simulink model "trainn_traction_system_4motors_CRH3_ver1"  (R2020b)
settings: Solver=VariableStepAuto  StartTime=0.0  StopTime=3  RelTol=1e-3
model workspace (MAT data in the model file):
  C = 0.016
  J = 5
  L = 0.005
  Llr = 0.006
  Lls = 0.001416
  Lm = 0.0254
  R = 0.2
  Rr = 0.16
  Rs = 0.15
  T = 1e-06
  Tloadmax = 100
  Tloadstart = 2
  Tpwm = 0.0001
  Ts = 0.0008
  Vdc_ref = 2700
  Vpeak = 1550
  f = 50
  noiseDense = 0.01
  np = 2
  sample_time = 2e-05
  tE1 = 3.25
  tE1w = 10
  tE2 = 10
  tE2w = 10
  tE3 = 10
  tE3w = 10
  tE4 = 10
  tE4w = 10
  t_precharge = 0.15
  w = 314.159265359
libraries: powerlib x19, simulink x19, pid_lib x1, eeSinusoidalMeasurementV2 x1
(part 2 of 3)

== system trainn_traction_system_4motors_CRH3_ver1/motor module2/Subsystem2/转矩调节器ATR ==
  " " : Inport
  Integrator : Integrator
  I积分放大倍数 : Gain  Gain=1.1
  PI输出限幅1 : Saturate  UpperLimit=600  LowerLimit=-600
  P比例放大倍数 : Gain  Gain=1.6
  Scope : Scope  NumInputPorts=2
  Sum3 : Sum  Inputs=|++
  带限幅的连续积分1 : Integrator  LimitOutput=on  UpperSaturationLimit=65  LowerSaturationLimit=-65
  ist* : Outport  VectorParamsAs1DForOutWhenUnconnected=off
  wires:
  " "/1 -> I积分放大倍数/1, P比例放大倍数/1
  I积分放大倍数/1 -> Integrator/1
  Sum3/1 -> PI输出限幅1/1
  P比例放大倍数/1 -> Sum3/1
  Integrator/1 -> Scope/2, Sum3/2
  PI输出限幅1/1 -> Scope/1, ist*/1

== system trainn_traction_system_4motors_CRH3_ver1/motor module2/Subsystem2/转速调节器ASR ==
  "  " : Inport
  Integrator : Integrator
  I积分放大倍数 : Gain  Gain=0.08
  PI输出限幅2 : Saturate  UpperLimit=400  LowerLimit=-400
  P比例放大倍数 : Gain  Gain=12
  Scope : Scope  NumInputPorts=2
  Sum1 : Sum  Inputs=|++
  带限幅的连续积分1 : Integrator  LimitOutput=on  UpperSaturationLimit=80  LowerSaturationLimit=-80
  Te* : Outport  VectorParamsAs1DForOutWhenUnconnected=off
  wires:
  I积分放大倍数/1 -> Integrator/1
  "  "/1 -> I积分放大倍数/1, P比例放大倍数/1
  P比例放大倍数/1 -> Sum1/1
  Integrator/1 -> Scope/2, Sum1/2
  Sum1/1 -> PI输出限幅2/1
  PI输出限幅2/1 -> Scope/1, Te*/1

== system trainn_traction_system_4motors_CRH3_ver1/motor module3/Subsystem3/ACMR ==
  "  " : Inport
  Integrator : Integrator
  I积分放大倍数 : Gain  Gain=50
  PI输出限幅 : Saturate  UpperLimit=Vdc_ref/sqrt(6)  LowerLimit=-Vdc_ref/sqrt(6)
  P比例放大倍数 : Gain
  Scope : Scope  NumInputPorts=2
  Sum1 : Sum  Inputs=|++
  带限幅的连续积分1 : Integrator  LimitOutput=on  UpperSaturationLimit=390  LowerSaturationLimit=-390
  " " : Outport  VectorParamsAs1DForOutWhenUnconnected=off
  wires:
  Sum1/1 -> PI输出限幅/1
  PI输出限幅/1 -> " "/1, Scope/1
  P比例放大倍数/1 -> Sum1/1
  I积分放大倍数/1 -> Integrator/1
  "  "/1 -> I积分放大倍数/1, P比例放大倍数/1
  Integrator/1 -> Scope/2, Sum1/2

== system trainn_traction_system_4motors_CRH3_ver1/motor module3/Subsystem3/ACTR ==
  "  " : Inport
  Integrator : Integrator
  I积分放大倍数 : Gain  Gain=3.5
  PI输出限幅 : Saturate  UpperLimit=Vdc_ref/sqrt(6)  LowerLimit=-1*Vdc_ref/sqrt(6)
  PI输出限幅1 : Saturate  UpperLimit=Vdc_ref  LowerLimit=-1*Vdc_ref
  P比例放大倍数 : Gain  Gain=1.5
  Scope : Scope  NumInputPorts=2
  Sum1 : Sum  Inputs=|++
  带限幅的连续积分1 : Integrator  LimitOutput=on  UpperSaturationLimit=400  LowerSaturationLimit=-400
  " " : Outport  VectorParamsAs1DForOutWhenUnconnected=off
  wires:
  Sum1/1 -> PI输出限幅/1
  PI输出限幅/1 -> " "/1, Scope/1
  P比例放大倍数/1 -> Sum1/1
  I积分放大倍数/1 -> Integrator/1
  "  "/1 -> I积分放大倍数/1, P比例放大倍数/1
  Integrator/1 -> Scope/2, Sum1/2

== system trainn_traction_system_4motors_CRH3_ver1/motor module3/Subsystem3/SVPWM ==
  Udc : Inport
  Ualpha : Inport  Port=2
  Ubeta : Inport  Port=3
  " Gen Gate" : MATLAB Function  TreatAsAtomicUnit=on
  Clock : Clock
  Constant2 : Constant  Value=Ts
  Constant3 : Constant  Value=Ts
  Data Type Conversion : DataTypeConversion  OutDataTypeStr=boolean
  Delay{,1..4} (5 alike) : Delay  DelayLength=1  InitialCondition=0
  MATLAB Function1 : MATLAB Function  TreatAsAtomicUnit=on
  MATLAB Function3 : MATLAB Function  TreatAsAtomicUnit=on
  Pulse Generator : DiscretePulseGenerator  PulseType=Time based  Period=Ts
  Scope1 : Scope  NumInputPorts=3
  Scope3 : Scope
  find section1 : Subsystem
  g : Outport
  wires:
  Ualpha/1 -> find section1/1(Ualpha), MATLAB Function3/2(Ualpha)
  Pulse Generator/1 -> Data Type Conversion/1
  MATLAB Function1/2(newT0) -> " Gen Gate"/4(T0), Delay/1
  Delay1/1 -> MATLAB Function1/1(old_t0)
  MATLAB Function3/3(T2) -> Scope1/3, MATLAB Function1/6(T2)
  Ubeta/1 -> find section1/2(Ubeta), MATLAB Function3/3(Ubeta)
  find section1/1(section) -> MATLAB Function1/7(sec), MATLAB Function3/5(sec)
  Constant2/1 -> MATLAB Function3/4(Ts)
  MATLAB Function3/2(T1) -> Scope1/2, MATLAB Function1/5(T1)
  MATLAB Function1/1(new_t0) -> Scope3/1, Delay1/1, " Gen Gate"/2(t0)
  Clock/1 -> " Gen Gate"/1(t), MATLAB Function1/2(t)
  MATLAB Function3/1(T0) -> MATLAB Function1/4(T0), Scope1/1
  Constant3/1 -> " Gen Gate"/3(Ts)
  Udc/1 -> MATLAB Function3/1(Udc)
  " Gen Gate"/1(g) -> g/1
  Data Type Conversion/1 -> MATLAB Function1/3(trigger)
  MATLAB Function1/5(newSec) -> Delay2/1, " Gen Gate"/7(sec)
  Delay2/1 -> MATLAB Function1/11(oldSec)
  MATLAB Function1/4(newT2) -> Delay3/1, " Gen Gate"/6(T2)
  Delay3/1 -> MATLAB Function1/10(oldT2)
  MATLAB Function1/3(newT1) -> Delay4/1, " Gen Gate"/5(T1)
  Delay4/1 -> MATLAB Function1/9(oldT1)
  Delay/1 -> MATLAB Function1/8(oldT0)

== system trainn_traction_system_4motors_CRH3_ver1/motor module3/Subsystem3/SVPWM1 ==
  Udc : Inport
  Ualpha : Inport  Port=2
  Ubeta : Inport  Port=3
  Constant2 : Constant  Value=Tpwm
  Constant4 : Constant  Value=Tpwm
  MATLAB Function10 : MATLAB Function  TreatAsAtomicUnit=on
  MATLAB Function3 : MATLAB Function  TreatAsAtomicUnit=on
  Mux : Mux  Inputs=6
  Repeating Sequence1 : simulink/Sources/Repeating Sequence  rep_seq_t=[0 Tpwm]  rep_seq_y=[0 Tpwm]
  Scope1 : Scope  NumInputPorts=3
  find section1 : Subsystem
  g : Outport
  wires:
  Ualpha/1 -> find section1/1(Ualpha), MATLAB Function3/2(Ualpha)
  Ubeta/1 -> find section1/2(Ubeta), MATLAB Function3/3(Ubeta)
  Constant2/1 -> MATLAB Function3/4(Ts)
  MATLAB Function3/1(T0) -> Scope1/1
  Udc/1 -> MATLAB Function3/1(Udc)
  MATLAB Function3/2(T1) -> Scope1/2, MATLAB Function10/1(Ta)
  find section1/1(section) -> MATLAB Function10/4(section), MATLAB Function3/5(sec)
  Constant4/1 -> MATLAB Function10/3(Tpwm)
  Repeating Sequence1/1 -> MATLAB Function10/5(t)
  MATLAB Function3/3(T2) -> Scope1/3, MATLAB Function10/2(Tb)
  MATLAB Function10/6(gCN) -> Mux/6
  MATLAB Function10/5(gC) -> Mux/5
  MATLAB Function10/4(gBN) -> Mux/4
  MATLAB Function10/3(gB) -> Mux/3
  MATLAB Function10/2(gAN) -> Mux/2
  MATLAB Function10/1(gA) -> Mux/1
  Mux/1 -> g/1

== system trainn_traction_system_4motors_CRH3_ver1/motor module3/Subsystem3/Subsystem ==
  note: Tr = Lr / Rr
  note: phy_r
  note: ws
  note: w1
  id(im) : Inport
  iq(it) : Inport  Port=2
  w : Inport  Port=3
  Divide{,2..4} (4 alike) : Product  Inputs=/*
  Divide1 : Product  Inputs=*/
  Gain1 : Gain  Gain=Lm
  Gain2 : Gain  Gain=Lm
  Integrator1 : Integrator  InitialCondition=1e-5
  Integrator2 : Integrator
  Lr : Constant  Value=Llr + 1.5*Lm
  Rr : Constant  Value=Rr
  Scope3 : Scope  NumInputPorts=2
  Sum : Sum  Inputs=-+|
  Sum1 : Sum  Inputs=|++
  phi : Outport
  theta : Outport  Port=2
  wires:
  Divide/1 -> Sum1/1
  Divide3/1 -> Divide/2
  Sum/1 -> Integrator1/1
  iq(it)/1 -> Gain2/1, Scope3/2
  Sum1/1 -> Integrator2/1
  id(im)/1 -> Gain1/1, Scope3/1
  w/1 -> Sum1/2
  Integrator2/1 -> theta/1
  Lr/1 -> Divide1/1
  Rr/1 -> Divide1/2
  Divide2/1 -> Sum/2
  Gain1/1 -> Divide2/2
  Integrator1/1 -> Divide4/2, Divide/1, phi/1
  Divide4/1 -> Sum/1
  Divide1/1 -> Divide3/1, Divide2/1, Divide4/1
  Gain2/1 -> Divide3/2

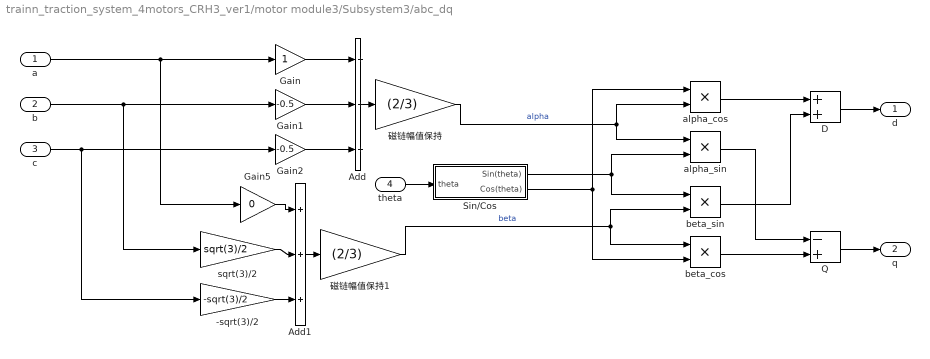
== system trainn_traction_system_4motors_CRH3_ver1/motor module3/Subsystem3/abc_dq ==
  a : Inport
  b : Inport  Port=2
  c : Inport  Port=3
  theta : Inport  Port=4
  -sqrt(3)/2 : Gain  Gain=-sqrt(3)/2
  Add : Sum  Inputs=3
  Add1 : Sum  Inputs=3
  D : Sum
  Gain : Gain
  Gain1 : Gain  Gain=-0.5
  Gain2 : Gain  Gain=-0.5
  Gain5 : Gain  Gain=0
  Q : Sum  Inputs=-+
  Sin/Cos : Subsystem
  alpha_cos : Product
  alpha_sin : Product
  beta_cos : Product
  beta_sin : Product
  sqrt(3)/2 : Gain  Gain=sqrt(3)/2
  磁链幅值保持 : Gain  Gain=(2/3)
  磁链幅值保持1 : Gain  Gain=(2/3)
  d : Outport  VectorParamsAs1DForOutWhenUnconnected=off
  q : Outport  Port=2  VectorParamsAs1DForOutWhenUnconnected=off
  wires:
  磁链幅值保持1/1 -> beta_cos/1, beta_sin/2  "beta"
  D/1 -> d/1
  Sin/Cos/2(Cos(theta)) -> beta_cos/2, alpha_cos/1
  alpha_sin/1 -> Q/1
  Q/1 -> q/1
  beta_sin/1 -> D/2
  beta_cos/1 -> Q/2
  Sin/Cos/1(Sin(theta)) -> beta_sin/1, alpha_sin/2
  磁链幅值保持/1 -> alpha_cos/2, alpha_sin/1  "alpha"
  Add1/1 -> 磁链幅值保持1/1
  c/1 -> Gain2/1, -sqrt(3)/2/1
  a/1 -> Gain5/1, Gain/1
  Gain2/1 -> Add/3
  sqrt(3)/2/1 -> Add1/2
  theta/1 -> Sin/Cos/1(theta)
  b/1 -> sqrt(3)/2/1, Gain1/1
  -sqrt(3)/2/1 -> Add1/3
  Gain1/1 -> Add/2
  Gain5/1 -> Add1/1
  alpha_cos/1 -> D/1
  Add/1 -> 磁链幅值保持/1
  Gain/1 -> Add/1

== system trainn_traction_system_4motors_CRH3_ver1/motor module3/Subsystem3/dq-alpha\beta1 ==
  Q : Inport
  D : Inport  Port=2
  theta : Inport  Port=3
  Product{,1..3} (4 alike) : Product
  Sum1 : Sum  Inputs=++|
  Sum3 : Sum  Inputs=|+-
  Trigonometric Function : Trigonometry
  Trigonometric Function1 : Trigonometry  Operator=cos
  alpha : Outport
  beta : Outport  Port=2
  wires:
  Sum1/1 -> beta/1
  Product3/1 -> Sum1/2
  Product2/1 -> Sum1/1
  Sum3/1 -> alpha/1
  Product1/1 -> Sum3/2
  Product/1 -> Sum3/1
  Trigonometric Function/1 -> Product1/1, Product2/1
  Trigonometric Function1/1 -> Product/2, Product3/1
  Q/1 -> Product1/2, Product3/2
  theta/1 -> Trigonometric Function/1, Trigonometric Function1/1
  D/1 -> Product2/2, Product/1

== system trainn_traction_system_4motors_CRH3_ver1/motor module3/Subsystem3/磁链调节器APhirR ==
  " " : Inport
  Integrator : Integrator
  I积分放大倍数 : Gain  Gain=3.6
  PI输出限幅1 : Saturate  UpperLimit=13  LowerLimit=-13
  P比例放大倍数 : Gain  Gain=1.8
  Scope : Scope  NumInputPorts=2
  Sum1 : Sum  Inputs=|++
  带限幅的连续积分1 : Integrator  LimitOutput=on  UpperSaturationLimit=15  LowerSaturationLimit=-15
  ism* : Outport  VectorParamsAs1DForOutWhenUnconnected=off
  wires:
  P比例放大倍数/1 -> Sum1/1
  " "/1 -> I积分放大倍数/1, P比例放大倍数/1
  Sum1/1 -> ism*/1, Scope/1
  I积分放大倍数/1 -> Integrator/1
  Integrator/1 -> Scope/2, Sum1/2

== system trainn_traction_system_4motors_CRH3_ver1/motor module3/Subsystem3/转矩调节器ATR ==
  " " : Inport
  Integrator : Integrator
  I积分放大倍数 : Gain  Gain=1.1
  PI输出限幅1 : Saturate  UpperLimit=600  LowerLimit=-600
  P比例放大倍数 : Gain  Gain=1.6
  Scope : Scope  NumInputPorts=2
  Sum3 : Sum  Inputs=|++
  带限幅的连续积分1 : Integrator  LimitOutput=on  UpperSaturationLimit=65  LowerSaturationLimit=-65
  ist* : Outport  VectorParamsAs1DForOutWhenUnconnected=off
  wires:
  " "/1 -> I积分放大倍数/1, P比例放大倍数/1
  I积分放大倍数/1 -> Integrator/1
  Sum3/1 -> PI输出限幅1/1
  P比例放大倍数/1 -> Sum3/1
  Integrator/1 -> Scope/2, Sum3/2
  PI输出限幅1/1 -> Scope/1, ist*/1

== system trainn_traction_system_4motors_CRH3_ver1/motor module3/Subsystem3/转速调节器ASR ==
  "  " : Inport
  Integrator : Integrator
  I积分放大倍数 : Gain  Gain=0.08
  PI输出限幅2 : Saturate  UpperLimit=400  LowerLimit=-400
  P比例放大倍数 : Gain  Gain=12
  Scope : Scope  NumInputPorts=2
  Sum1 : Sum  Inputs=|++
  带限幅的连续积分1 : Integrator  LimitOutput=on  UpperSaturationLimit=80  LowerSaturationLimit=-80
  Te* : Outport  VectorParamsAs1DForOutWhenUnconnected=off
  wires:
  I积分放大倍数/1 -> Integrator/1
  "  "/1 -> I积分放大倍数/1, P比例放大倍数/1
  P比例放大倍数/1 -> Sum1/1
  Integrator/1 -> Scope/2, Sum1/2
  Sum1/1 -> PI输出限幅2/1
  PI输出限幅2/1 -> Scope/1, Te*/1

== system trainn_traction_system_4motors_CRH3_ver1/motor module4/电机控制模块/ACMR ==
  "  " : Inport
  Integrator : Integrator
  I积分放大倍数 : Gain  Gain=50
  PI输出限幅 : Saturate  UpperLimit=Vdc_ref/sqrt(6)  LowerLimit=-Vdc_ref/sqrt(6)
  P比例放大倍数 : Gain
  Scope : Scope  NumInputPorts=2
  Sum1 : Sum  Inputs=|++
  带限幅的连续积分1 : Integrator  LimitOutput=on  UpperSaturationLimit=390  LowerSaturationLimit=-390
  " " : Outport  VectorParamsAs1DForOutWhenUnconnected=off
  wires:
  Integrator/1 -> Sum1/2, Scope/2
  "  "/1 -> P比例放大倍数/1, I积分放大倍数/1
  I积分放大倍数/1 -> Integrator/1
  P比例放大倍数/1 -> Sum1/1
  PI输出限幅/1 -> Scope/1, " "/1
  Sum1/1 -> PI输出限幅/1

== system trainn_traction_system_4motors_CRH3_ver1/motor module4/电机控制模块/ACTR ==
  "  " : Inport
  Integrator : Integrator
  I积分放大倍数 : Gain  Gain=3.5
  PI输出限幅 : Saturate  UpperLimit=Vdc_ref/sqrt(6)  LowerLimit=-1*Vdc_ref/sqrt(6)
  PI输出限幅1 : Saturate  UpperLimit=Vdc_ref  LowerLimit=-1*Vdc_ref
  P比例放大倍数 : Gain  Gain=1.5
  Scope : Scope  NumInputPorts=2
  Sum1 : Sum  Inputs=|++
  带限幅的连续积分1 : Integrator  LimitOutput=on  UpperSaturationLimit=400  LowerSaturationLimit=-400
  " " : Outport  VectorParamsAs1DForOutWhenUnconnected=off
  wires:
  Integrator/1 -> Sum1/2, Scope/2
  "  "/1 -> P比例放大倍数/1, I积分放大倍数/1
  I积分放大倍数/1 -> Integrator/1
  P比例放大倍数/1 -> Sum1/1
  PI输出限幅/1 -> Scope/1, " "/1
  Sum1/1 -> PI输出限幅/1

== system trainn_traction_system_4motors_CRH3_ver1/motor module4/电机控制模块/SVPWM ==
  Udc : Inport
  Ualpha : Inport  Port=2
  Ubeta : Inport  Port=3
  " Gen Gate" : MATLAB Function  TreatAsAtomicUnit=on
  Clock : Clock
  Constant2 : Constant  Value=Ts
  Constant3 : Constant  Value=Ts
  Data Type Conversion : DataTypeConversion  OutDataTypeStr=boolean
  Delay{,1..4} (5 alike) : Delay  DelayLength=1  InitialCondition=0
  MATLAB Function1 : MATLAB Function  TreatAsAtomicUnit=on
  MATLAB Function3 : MATLAB Function  TreatAsAtomicUnit=on
  Pulse Generator : DiscretePulseGenerator  PulseType=Time based  Period=Ts
  Scope1 : Scope  NumInputPorts=3
  Scope3 : Scope
  find section1 : Subsystem
  g : Outport
  wires:
  Delay/1 -> MATLAB Function1/8(oldT0)
  Delay4/1 -> MATLAB Function1/9(oldT1)
  MATLAB Function1/3(newT1) -> " Gen Gate"/5(T1), Delay4/1
  Delay3/1 -> MATLAB Function1/10(oldT2)
  MATLAB Function1/4(newT2) -> " Gen Gate"/6(T2), Delay3/1
  Delay2/1 -> MATLAB Function1/11(oldSec)
  MATLAB Function1/5(newSec) -> " Gen Gate"/7(sec), Delay2/1
  Data Type Conversion/1 -> MATLAB Function1/3(trigger)
  " Gen Gate"/1(g) -> g/1
  Udc/1 -> MATLAB Function3/1(Udc)
  Constant3/1 -> " Gen Gate"/3(Ts)
  MATLAB Function3/1(T0) -> Scope1/1, MATLAB Function1/4(T0)
  Clock/1 -> MATLAB Function1/2(t), " Gen Gate"/1(t)
  MATLAB Function1/1(new_t0) -> " Gen Gate"/2(t0), Delay1/1, Scope3/1
  MATLAB Function3/2(T1) -> MATLAB Function1/5(T1), Scope1/2
  Constant2/1 -> MATLAB Function3/4(Ts)
  find section1/1(section) -> MATLAB Function3/5(sec), MATLAB Function1/7(sec)
  Ubeta/1 -> MATLAB Function3/3(Ubeta), find section1/2(Ubeta)
  MATLAB Function3/3(T2) -> MATLAB Function1/6(T2), Scope1/3
  Delay1/1 -> MATLAB Function1/1(old_t0)
  MATLAB Function1/2(newT0) -> Delay/1, " Gen Gate"/4(T0)
  Pulse Generator/1 -> Data Type Conversion/1
  Ualpha/1 -> MATLAB Function3/2(Ualpha), find section1/1(Ualpha)

== system trainn_traction_system_4motors_CRH3_ver1/motor module4/电机控制模块/SVPWM1 ==
  Udc : Inport
  Ualpha : Inport  Port=2
  Ubeta : Inport  Port=3
  Constant2 : Constant  Value=Tpwm
  Constant4 : Constant  Value=Tpwm
  MATLAB Function10 : MATLAB Function  TreatAsAtomicUnit=on
  MATLAB Function3 : MATLAB Function  TreatAsAtomicUnit=on
  Mux : Mux  Inputs=6
  Repeating Sequence1 : simulink/Sources/Repeating Sequence  rep_seq_t=[0 Tpwm]  rep_seq_y=[0 Tpwm]
  Scope1 : Scope  NumInputPorts=3
  find section1 : Subsystem
  g : Outport
  wires:
  Ualpha/1 -> find section1/1(Ualpha), MATLAB Function3/2(Ualpha)
  Ubeta/1 -> find section1/2(Ubeta), MATLAB Function3/3(Ubeta)
  Constant2/1 -> MATLAB Function3/4(Ts)
  MATLAB Function3/1(T0) -> Scope1/1
  Udc/1 -> MATLAB Function3/1(Udc)
  MATLAB Function3/2(T1) -> Scope1/2, MATLAB Function10/1(Ta)
  find section1/1(section) -> MATLAB Function10/4(section), MATLAB Function3/5(sec)
  Constant4/1 -> MATLAB Function10/3(Tpwm)
  Repeating Sequence1/1 -> MATLAB Function10/5(t)
  MATLAB Function3/3(T2) -> Scope1/3, MATLAB Function10/2(Tb)
  MATLAB Function10/6(gCN) -> Mux/6
  MATLAB Function10/5(gC) -> Mux/5
  MATLAB Function10/4(gBN) -> Mux/4
  MATLAB Function10/3(gB) -> Mux/3
  MATLAB Function10/2(gAN) -> Mux/2
  MATLAB Function10/1(gA) -> Mux/1
  Mux/1 -> g/1

== system trainn_traction_system_4motors_CRH3_ver1/motor module4/电机控制模块/Subsystem ==
  note: w1
  note: ws
  note: phy_r
  note: Tr = Lr / Rr
  id(im) : Inport
  iq(it) : Inport  Port=2
  w : Inport  Port=3
  Divide{,2..4} (4 alike) : Product  Inputs=/*
  Divide1 : Product  Inputs=*/
  Gain1 : Gain  Gain=Lm
  Gain2 : Gain  Gain=Lm
  Integrator1 : Integrator  InitialCondition=1e-5
  Integrator2 : Integrator
  Lr : Constant  Value=Llr + 1.5*Lm
  Rr : Constant  Value=Rr
  Scope3 : Scope  NumInputPorts=2
  Sum : Sum  Inputs=-+|
  Sum1 : Sum  Inputs=|++
  phi : Outport
  theta : Outport  Port=2
  wires:
  Gain2/1 -> Divide3/2
  Divide1/1 -> Divide4/1, Divide2/1, Divide3/1
  Divide4/1 -> Sum/1
  Integrator1/1 -> phi/1, Divide/1, Divide4/2
  Gain1/1 -> Divide2/2
  Divide2/1 -> Sum/2
  Rr/1 -> Divide1/2
  Lr/1 -> Divide1/1
  Integrator2/1 -> theta/1
  w/1 -> Sum1/2
  id(im)/1 -> Scope3/1, Gain1/1
  Sum1/1 -> Integrator2/1
  iq(it)/1 -> Scope3/2, Gain2/1
  Sum/1 -> Integrator1/1
  Divide3/1 -> Divide/2
  Divide/1 -> Sum1/1

== system trainn_traction_system_4motors_CRH3_ver1/motor module4/电机控制模块/abc_dq ==
  a : Inport
  b : Inport  Port=2
  c : Inport  Port=3
  theta : Inport  Port=4
  -sqrt(3)/2 : Gain  Gain=-sqrt(3)/2
  Add : Sum  Inputs=3
  Add1 : Sum  Inputs=3
  D : Sum
  Gain : Gain
  Gain1 : Gain  Gain=-0.5
  Gain2 : Gain  Gain=-0.5
  Gain5 : Gain  Gain=0
  Q : Sum  Inputs=-+
  Sin/Cos : Subsystem
  alpha_cos : Product
  alpha_sin : Product
  beta_cos : Product
  beta_sin : Product
  sqrt(3)/2 : Gain  Gain=sqrt(3)/2
  磁链幅值保持 : Gain  Gain=(2/3)
  磁链幅值保持1 : Gain  Gain=(2/3)
  d : Outport  VectorParamsAs1DForOutWhenUnconnected=off
  q : Outport  Port=2  VectorParamsAs1DForOutWhenUnconnected=off
  wires:
  Gain/1 -> Add/1
  Add/1 -> 磁链幅值保持/1
  alpha_cos/1 -> D/1
  Gain5/1 -> Add1/1
  Gain1/1 -> Add/2
  -sqrt(3)/2/1 -> Add1/3
  b/1 -> Gain1/1, sqrt(3)/2/1
  theta/1 -> Sin/Cos/1(theta)
  sqrt(3)/2/1 -> Add1/2
  Gain2/1 -> Add/3
  a/1 -> Gain/1, Gain5/1
  c/1 -> -sqrt(3)/2/1, Gain2/1
  Add1/1 -> 磁链幅值保持1/1
  磁链幅值保持/1 -> alpha_sin/1, alpha_cos/2  "alpha"
  Sin/Cos/1(Sin(theta)) -> alpha_sin/2, beta_sin/1
  beta_cos/1 -> Q/2
  beta_sin/1 -> D/2
  Q/1 -> q/1
  alpha_sin/1 -> Q/1
  Sin/Cos/2(Cos(theta)) -> alpha_cos/1, beta_cos/2
  D/1 -> d/1
  磁链幅值保持1/1 -> beta_sin/2, beta_cos/1  "beta"

== system trainn_traction_system_4motors_CRH3_ver1/motor module4/电机控制模块/dq-alpha\beta1 ==
  Q : Inport
  D : Inport  Port=2
  theta : Inport  Port=3
  Product{,1..3} (4 alike) : Product
  Sum1 : Sum  Inputs=++|
  Sum3 : Sum  Inputs=|+-
  Trigonometric Function : Trigonometry
  Trigonometric Function1 : Trigonometry  Operator=cos
  alpha : Outport
  beta : Outport  Port=2
  wires:
  D/1 -> Product/1, Product2/2
  theta/1 -> Trigonometric Function1/1, Trigonometric Function/1
  Q/1 -> Product3/2, Product1/2
  Trigonometric Function1/1 -> Product3/1, Product/2
  Trigonometric Function/1 -> Product2/1, Product1/1
  Product/1 -> Sum3/1
  Product1/1 -> Sum3/2
  Sum3/1 -> alpha/1
  Product2/1 -> Sum1/1
  Product3/1 -> Sum1/2
  Sum1/1 -> beta/1

== system trainn_traction_system_4motors_CRH3_ver1/motor module4/电机控制模块/磁链调节器APhirR ==
  " " : Inport
  Integrator : Integrator
  I积分放大倍数 : Gain  Gain=3.6
  PI输出限幅1 : Saturate  UpperLimit=13  LowerLimit=-13
  P比例放大倍数 : Gain  Gain=1.8
  Scope : Scope  NumInputPorts=2
  Sum1 : Sum  Inputs=|++
  带限幅的连续积分1 : Integrator  LimitOutput=on  UpperSaturationLimit=15  LowerSaturationLimit=-15
  ism* : Outport  VectorParamsAs1DForOutWhenUnconnected=off
  wires:
  Integrator/1 -> Sum1/2, Scope/2
  I积分放大倍数/1 -> Integrator/1
  Sum1/1 -> Scope/1, ism*/1
  " "/1 -> P比例放大倍数/1, I积分放大倍数/1
  P比例放大倍数/1 -> Sum1/1

== system trainn_traction_system_4motors_CRH3_ver1/motor module4/电机控制模块/转矩调节器ATR ==
  " " : Inport
  Integrator : Integrator
  I积分放大倍数 : Gain  Gain=1.1
  PI输出限幅1 : Saturate  UpperLimit=600  LowerLimit=-600
  P比例放大倍数 : Gain  Gain=1.6
  Scope : Scope  NumInputPorts=2
  Sum3 : Sum  Inputs=|++
  带限幅的连续积分1 : Integrator  LimitOutput=on  UpperSaturationLimit=65  LowerSaturationLimit=-65
  ist* : Outport  VectorParamsAs1DForOutWhenUnconnected=off
  wires:
  " "/1 -> I积分放大倍数/1, P比例放大倍数/1
  I积分放大倍数/1 -> Integrator/1
  Sum3/1 -> PI输出限幅1/1
  P比例放大倍数/1 -> Sum3/1
  Integrator/1 -> Scope/2, Sum3/2
  PI输出限幅1/1 -> Scope/1, ist*/1

== system trainn_traction_system_4motors_CRH3_ver1/motor module4/电机控制模块/转速调节器ASR ==
  "  " : Inport
  Integrator : Integrator
  I积分放大倍数 : Gain  Gain=0.08
  PI输出限幅2 : Saturate  UpperLimit=400  LowerLimit=-400
  P比例放大倍数 : Gain  Gain=12
  Scope : Scope  NumInputPorts=2
  Sum1 : Sum  Inputs=|++
  带限幅的连续积分1 : Integrator  LimitOutput=on  UpperSaturationLimit=80  LowerSaturationLimit=-80
  Te* : Outport  VectorParamsAs1DForOutWhenUnconnected=off
  wires:
  I积分放大倍数/1 -> Integrator/1
  "  "/1 -> I积分放大倍数/1, P比例放大倍数/1
  P比例放大倍数/1 -> Sum1/1
  Integrator/1 -> Scope/2, Sum1/2
  Sum1/1 -> PI输出限幅2/1
  PI输出限幅2/1 -> Scope/1, Te*/1

== system trainn_traction_system_4motors_CRH3_ver1/motor module1/Subsystem1/SVPWM/find section1 ==
  Ualpha : Inport
  Ubeta : Inport  Port=2
  >=0? : Subsystem
  Gain : Gain  Gain=sqrt(3)
  Gain1 : Gain  Gain=4
  Gain2 : Gain  Gain=2
  Sum : Sum  Inputs=++|
  Sum1 : Sum  Inputs=-+|
  Sum2 : Sum  Inputs=+++
  get section : MATLAB Function  TreatAsAtomicUnit=on
  not neg : Subsystem
  not neg1 : Subsystem
  section : Outport
  wires:
  Gain2/1 -> Sum2/2
  get section/1(y) -> section/1
  Ubeta/1 -> >=0?/1(In1), Sum1/2, Sum/2
  Gain/1 -> Sum1/1, Sum/1
  Gain1/1 -> Sum2/3
  Sum1/1 -> not neg/1(In1)
  Sum/1 -> not neg1/1(In1)
  >=0?/1(Out1) -> Gain1/1
  not neg1/1(Out1) -> Sum2/1
  Sum2/1 -> get section/1(u)
  not neg/1(Out1) -> Gain2/1
  Ualpha/1 -> Gain/1

== system trainn_traction_system_4motors_CRH3_ver1/motor module1/Subsystem1/SVPWM1/find section1 ==
  Ualpha : Inport
  Ubeta : Inport  Port=2
  >=0? : Subsystem
  Gain : Gain  Gain=sqrt(3)
  Gain1 : Gain  Gain=4
  Gain2 : Gain  Gain=2
  Sum : Sum  Inputs=++|
  Sum1 : Sum  Inputs=-+|
  Sum2 : Sum  Inputs=+++
  get section : MATLAB Function  TreatAsAtomicUnit=on
  not neg : Subsystem
  not neg1 : Subsystem
  section : Outport
  wires:
  Gain2/1 -> Sum2/2
  get section/1(y) -> section/1
  Ubeta/1 -> >=0?/1(In1), Sum1/2, Sum/2
  Gain/1 -> Sum1/1, Sum/1
  Gain1/1 -> Sum2/3
  Sum1/1 -> not neg/1(In1)
  Sum/1 -> not neg1/1(In1)
  >=0?/1(Out1) -> Gain1/1
  not neg1/1(Out1) -> Sum2/1
  Sum2/1 -> get section/1(u)
  not neg/1(Out1) -> Gain2/1
  Ualpha/1 -> Gain/1

== system trainn_traction_system_4motors_CRH3_ver1/motor module1/Subsystem1/abc_dq/Sin//Cos ==
  theta : Inport
  cos : Trigonometry  Operator=cos
  sin : Trigonometry
  Sin(theta) : Outport  VectorParamsAs1DForOutWhenUnconnected=off
  Cos(theta) : Outport  Port=2  VectorParamsAs1DForOutWhenUnconnected=off
  wires:
  sin/1 -> Sin(theta)/1
  theta/1 -> sin/1, cos/1
  cos/1 -> Cos(theta)/1

== system trainn_traction_system_4motors_CRH3_ver1/motor module2/Subsystem2/SVPWM/find section1 ==
  Ualpha : Inport
  Ubeta : Inport  Port=2
  >=0? : Subsystem
  Gain : Gain  Gain=sqrt(3)
  Gain1 : Gain  Gain=4
  Gain2 : Gain  Gain=2
  Sum : Sum  Inputs=++|
  Sum1 : Sum  Inputs=-+|
  Sum2 : Sum  Inputs=+++
  get section : MATLAB Function  TreatAsAtomicUnit=on
  not neg : Subsystem
  not neg1 : Subsystem
  section : Outport
  wires:
  Gain2/1 -> Sum2/2
  get section/1(y) -> section/1
  Ubeta/1 -> >=0?/1(In1), Sum1/2, Sum/2
  Gain/1 -> Sum1/1, Sum/1
  Gain1/1 -> Sum2/3
  Sum1/1 -> not neg/1(In1)
  Sum/1 -> not neg1/1(In1)
  >=0?/1(Out1) -> Gain1/1
  not neg1/1(Out1) -> Sum2/1
  Sum2/1 -> get section/1(u)
  not neg/1(Out1) -> Gain2/1
  Ualpha/1 -> Gain/1

== system trainn_traction_system_4motors_CRH3_ver1/motor module2/Subsystem2/SVPWM1/find section1 ==
  Ualpha : Inport
  Ubeta : Inport  Port=2
  >=0? : Subsystem
  Gain : Gain  Gain=sqrt(3)
  Gain1 : Gain  Gain=4
  Gain2 : Gain  Gain=2
  Sum : Sum  Inputs=++|
  Sum1 : Sum  Inputs=-+|
  Sum2 : Sum  Inputs=+++
  get section : MATLAB Function  TreatAsAtomicUnit=on
  not neg : Subsystem
  not neg1 : Subsystem
  section : Outport
  wires:
  Gain2/1 -> Sum2/2
  get section/1(y) -> section/1
  Ubeta/1 -> >=0?/1(In1), Sum1/2, Sum/2
  Gain/1 -> Sum1/1, Sum/1
  Gain1/1 -> Sum2/3
  Sum1/1 -> not neg/1(In1)
  Sum/1 -> not neg1/1(In1)
  >=0?/1(Out1) -> Gain1/1
  not neg1/1(Out1) -> Sum2/1
  Sum2/1 -> get section/1(u)
  not neg/1(Out1) -> Gain2/1
  Ualpha/1 -> Gain/1

== system trainn_traction_system_4motors_CRH3_ver1/motor module2/Subsystem2/abc_dq/Sin//Cos ==
  theta : Inport
  cos : Trigonometry  Operator=cos
  sin : Trigonometry
  Sin(theta) : Outport  VectorParamsAs1DForOutWhenUnconnected=off
  Cos(theta) : Outport  Port=2  VectorParamsAs1DForOutWhenUnconnected=off
  wires:
  sin/1 -> Sin(theta)/1
  theta/1 -> sin/1, cos/1
  cos/1 -> Cos(theta)/1

== system trainn_traction_system_4motors_CRH3_ver1/motor module3/Subsystem3/SVPWM/find section1 ==
  Ualpha : Inport
  Ubeta : Inport  Port=2
  >=0? : Subsystem
  Gain : Gain  Gain=sqrt(3)
  Gain1 : Gain  Gain=4
  Gain2 : Gain  Gain=2
  Sum : Sum  Inputs=++|
  Sum1 : Sum  Inputs=-+|
  Sum2 : Sum  Inputs=+++
  get section : MATLAB Function  TreatAsAtomicUnit=on
  not neg : Subsystem
  not neg1 : Subsystem
  section : Outport
  wires:
  Gain2/1 -> Sum2/2
  get section/1(y) -> section/1
  Ubeta/1 -> >=0?/1(In1), Sum1/2, Sum/2
  Gain/1 -> Sum1/1, Sum/1
  Gain1/1 -> Sum2/3
  Sum1/1 -> not neg/1(In1)
  Sum/1 -> not neg1/1(In1)
  >=0?/1(Out1) -> Gain1/1
  not neg1/1(Out1) -> Sum2/1
  Sum2/1 -> get section/1(u)
  not neg/1(Out1) -> Gain2/1
  Ualpha/1 -> Gain/1

== system trainn_traction_system_4motors_CRH3_ver1/motor module3/Subsystem3/SVPWM1/find section1 ==
  Ualpha : Inport
  Ubeta : Inport  Port=2
  >=0? : Subsystem
  Gain : Gain  Gain=sqrt(3)
  Gain1 : Gain  Gain=4
  Gain2 : Gain  Gain=2
  Sum : Sum  Inputs=++|
  Sum1 : Sum  Inputs=-+|
  Sum2 : Sum  Inputs=+++
  get section : MATLAB Function  TreatAsAtomicUnit=on
  not neg : Subsystem
  not neg1 : Subsystem
  section : Outport
  wires:
  Gain2/1 -> Sum2/2
  get section/1(y) -> section/1
  Ubeta/1 -> >=0?/1(In1), Sum1/2, Sum/2
  Gain/1 -> Sum1/1, Sum/1
  Gain1/1 -> Sum2/3
  Sum1/1 -> not neg/1(In1)
  Sum/1 -> not neg1/1(In1)
  >=0?/1(Out1) -> Gain1/1
  not neg1/1(Out1) -> Sum2/1
  Sum2/1 -> get section/1(u)
  not neg/1(Out1) -> Gain2/1
  Ualpha/1 -> Gain/1

== system trainn_traction_system_4motors_CRH3_ver1/motor module3/Subsystem3/abc_dq/Sin//Cos ==
  theta : Inport
  cos : Trigonometry  Operator=cos
  sin : Trigonometry
  Sin(theta) : Outport  VectorParamsAs1DForOutWhenUnconnected=off
  Cos(theta) : Outport  Port=2  VectorParamsAs1DForOutWhenUnconnected=off
  wires:
  sin/1 -> Sin(theta)/1
  theta/1 -> sin/1, cos/1
  cos/1 -> Cos(theta)/1

== system trainn_traction_system_4motors_CRH3_ver1/motor module4/电机控制模块/SVPWM/find section1 ==
  Ualpha : Inport
  Ubeta : Inport  Port=2
  >=0? : Subsystem
  Gain : Gain  Gain=sqrt(3)
  Gain1 : Gain  Gain=4
  Gain2 : Gain  Gain=2
  Sum : Sum  Inputs=++|
  Sum1 : Sum  Inputs=-+|
  Sum2 : Sum  Inputs=+++
  get section : MATLAB Function  TreatAsAtomicUnit=on
  not neg : Subsystem
  not neg1 : Subsystem
  section : Outport
  wires:
  Ualpha/1 -> Gain/1
  not neg/1(Out1) -> Gain2/1
  Sum2/1 -> get section/1(u)
  not neg1/1(Out1) -> Sum2/1
  >=0?/1(Out1) -> Gain1/1
  Sum/1 -> not neg1/1(In1)
  Sum1/1 -> not neg/1(In1)
  Gain1/1 -> Sum2/3
  Gain/1 -> Sum/1, Sum1/1
  Ubeta/1 -> Sum/2, Sum1/2, >=0?/1(In1)
  get section/1(y) -> section/1
  Gain2/1 -> Sum2/2

== system trainn_traction_system_4motors_CRH3_ver1/motor module4/电机控制模块/SVPWM1/find section1 ==
  Ualpha : Inport
  Ubeta : Inport  Port=2
  >=0? : Subsystem
  Gain : Gain  Gain=sqrt(3)
  Gain1 : Gain  Gain=4
  Gain2 : Gain  Gain=2
  Sum : Sum  Inputs=++|
  Sum1 : Sum  Inputs=-+|
  Sum2 : Sum  Inputs=+++
  get section : MATLAB Function  TreatAsAtomicUnit=on
  not neg : Subsystem
  not neg1 : Subsystem
  section : Outport
  wires:
  Gain2/1 -> Sum2/2
  get section/1(y) -> section/1
  Ubeta/1 -> >=0?/1(In1), Sum1/2, Sum/2
  Gain/1 -> Sum1/1, Sum/1
  Gain1/1 -> Sum2/3
  Sum1/1 -> not neg/1(In1)
  Sum/1 -> not neg1/1(In1)
  >=0?/1(Out1) -> Gain1/1
  not neg1/1(Out1) -> Sum2/1
  Sum2/1 -> get section/1(u)
  not neg/1(Out1) -> Gain2/1
  Ualpha/1 -> Gain/1

== system trainn_traction_system_4motors_CRH3_ver1/motor module4/电机控制模块/abc_dq/Sin//Cos ==
  theta : Inport
  cos : Trigonometry  Operator=cos
  sin : Trigonometry
  Sin(theta) : Outport  VectorParamsAs1DForOutWhenUnconnected=off
  Cos(theta) : Outport  Port=2  VectorParamsAs1DForOutWhenUnconnected=off
  wires:
  cos/1 -> Cos(theta)/1
  theta/1 -> cos/1, sin/1
  sin/1 -> Sin(theta)/1

== system trainn_traction_system_4motors_CRH3_ver1/motor module1/Subsystem1/SVPWM/find section1/>=0? ==
  In1 : Inport
  Constant2 : Constant  Value=0
  Relational Operator : RelationalOperator  OutDataTypeStr=boolean  RndMeth=Simplest
  Out1 : Outport
  wires:
  Constant2/1 -> Relational Operator/2
  Relational Operator/1 -> Out1/1
  In1/1 -> Relational Operator/1

== system trainn_traction_system_4motors_CRH3_ver1/motor module1/Subsystem1/SVPWM/find section1/not neg ==
  In1 : Inport
  Constant2 : Constant  Value=0
  Relational Operator : RelationalOperator  OutDataTypeStr=boolean  RndMeth=Simplest
  Out1 : Outport
  wires:
  In1/1 -> Relational Operator/1
  Relational Operator/1 -> Out1/1
  Constant2/1 -> Relational Operator/2

== system trainn_traction_system_4motors_CRH3_ver1/motor module1/Subsystem1/SVPWM/find section1/not neg1 ==
  In1 : Inport
  Constant2 : Constant  Value=0
  Relational Operator : RelationalOperator  OutDataTypeStr=boolean  RndMeth=Simplest
  Out1 : Outport
  wires:
  Constant2/1 -> Relational Operator/2
  Relational Operator/1 -> Out1/1
  In1/1 -> Relational Operator/1

== system trainn_traction_system_4motors_CRH3_ver1/motor module1/Subsystem1/SVPWM1/find section1/>=0? ==
  In1 : Inport
  Constant2 : Constant  Value=0
  Relational Operator : RelationalOperator  OutDataTypeStr=boolean  RndMeth=Simplest
  Out1 : Outport
  wires:
  Constant2/1 -> Relational Operator/2
  Relational Operator/1 -> Out1/1
  In1/1 -> Relational Operator/1

== system trainn_traction_system_4motors_CRH3_ver1/motor module1/Subsystem1/SVPWM1/find section1/not neg ==
  In1 : Inport
  Constant2 : Constant  Value=0
  Relational Operator : RelationalOperator  OutDataTypeStr=boolean  RndMeth=Simplest
  Out1 : Outport
  wires:
  In1/1 -> Relational Operator/1
  Relational Operator/1 -> Out1/1
  Constant2/1 -> Relational Operator/2

== system trainn_traction_system_4motors_CRH3_ver1/motor module1/Subsystem1/SVPWM1/find section1/not neg1 ==
  In1 : Inport
  Constant2 : Constant  Value=0
  Relational Operator : RelationalOperator  OutDataTypeStr=boolean  RndMeth=Simplest
  Out1 : Outport
  wires:
  Constant2/1 -> Relational Operator/2
  Relational Operator/1 -> Out1/1
  In1/1 -> Relational Operator/1

== system trainn_traction_system_4motors_CRH3_ver1/motor module2/Subsystem2/SVPWM/find section1/>=0? ==
  In1 : Inport
  Constant2 : Constant  Value=0
  Relational Operator : RelationalOperator  OutDataTypeStr=boolean  RndMeth=Simplest
  Out1 : Outport
  wires:
  Constant2/1 -> Relational Operator/2
  Relational Operator/1 -> Out1/1
  In1/1 -> Relational Operator/1

== system trainn_traction_system_4motors_CRH3_ver1/motor module2/Subsystem2/SVPWM/find section1/not neg ==
  In1 : Inport
  Constant2 : Constant  Value=0
  Relational Operator : RelationalOperator  OutDataTypeStr=boolean  RndMeth=Simplest
  Out1 : Outport
  wires:
  In1/1 -> Relational Operator/1
  Relational Operator/1 -> Out1/1
  Constant2/1 -> Relational Operator/2

== system trainn_traction_system_4motors_CRH3_ver1/motor module2/Subsystem2/SVPWM/find section1/not neg1 ==
  In1 : Inport
  Constant2 : Constant  Value=0
  Relational Operator : RelationalOperator  OutDataTypeStr=boolean  RndMeth=Simplest
  Out1 : Outport
  wires:
  Constant2/1 -> Relational Operator/2
  Relational Operator/1 -> Out1/1
  In1/1 -> Relational Operator/1

== system trainn_traction_system_4motors_CRH3_ver1/motor module2/Subsystem2/SVPWM1/find section1/>=0? ==
  In1 : Inport
  Constant2 : Constant  Value=0
  Relational Operator : RelationalOperator  OutDataTypeStr=boolean  RndMeth=Simplest
  Out1 : Outport
  wires:
  Constant2/1 -> Relational Operator/2
  Relational Operator/1 -> Out1/1
  In1/1 -> Relational Operator/1

== system trainn_traction_system_4motors_CRH3_ver1/motor module2/Subsystem2/SVPWM1/find section1/not neg ==
  In1 : Inport
  Constant2 : Constant  Value=0
  Relational Operator : RelationalOperator  OutDataTypeStr=boolean  RndMeth=Simplest
  Out1 : Outport
  wires:
  In1/1 -> Relational Operator/1
  Relational Operator/1 -> Out1/1
  Constant2/1 -> Relational Operator/2

== system trainn_traction_system_4motors_CRH3_ver1/motor module2/Subsystem2/SVPWM1/find section1/not neg1 ==
  In1 : Inport
  Constant2 : Constant  Value=0
  Relational Operator : RelationalOperator  OutDataTypeStr=boolean  RndMeth=Simplest
  Out1 : Outport
  wires:
  Constant2/1 -> Relational Operator/2
  Relational Operator/1 -> Out1/1
  In1/1 -> Relational Operator/1

== system trainn_traction_system_4motors_CRH3_ver1/motor module3/Subsystem3/SVPWM/find section1/>=0? ==
  In1 : Inport
  Constant2 : Constant  Value=0
  Relational Operator : RelationalOperator  OutDataTypeStr=boolean  RndMeth=Simplest
  Out1 : Outport
  wires:
  Constant2/1 -> Relational Operator/2
  Relational Operator/1 -> Out1/1
  In1/1 -> Relational Operator/1

== system trainn_traction_system_4motors_CRH3_ver1/motor module3/Subsystem3/SVPWM/find section1/not neg ==
  In1 : Inport
  Constant2 : Constant  Value=0
  Relational Operator : RelationalOperator  OutDataTypeStr=boolean  RndMeth=Simplest
  Out1 : Outport
  wires:
  In1/1 -> Relational Operator/1
  Relational Operator/1 -> Out1/1
  Constant2/1 -> Relational Operator/2

== system trainn_traction_system_4motors_CRH3_ver1/motor module3/Subsystem3/SVPWM/find section1/not neg1 ==
  In1 : Inport
  Constant2 : Constant  Value=0
  Relational Operator : RelationalOperator  OutDataTypeStr=boolean  RndMeth=Simplest
  Out1 : Outport
  wires:
  Constant2/1 -> Relational Operator/2
  Relational Operator/1 -> Out1/1
  In1/1 -> Relational Operator/1

== system trainn_traction_system_4motors_CRH3_ver1/motor module3/Subsystem3/SVPWM1/find section1/>=0? ==
  In1 : Inport
  Constant2 : Constant  Value=0
  Relational Operator : RelationalOperator  OutDataTypeStr=boolean  RndMeth=Simplest
  Out1 : Outport
  wires:
  Constant2/1 -> Relational Operator/2
  Relational Operator/1 -> Out1/1
  In1/1 -> Relational Operator/1

== system trainn_traction_system_4motors_CRH3_ver1/motor module3/Subsystem3/SVPWM1/find section1/not neg ==
  In1 : Inport
  Constant2 : Constant  Value=0
  Relational Operator : RelationalOperator  OutDataTypeStr=boolean  RndMeth=Simplest
  Out1 : Outport
  wires:
  In1/1 -> Relational Operator/1
  Relational Operator/1 -> Out1/1
  Constant2/1 -> Relational Operator/2

== system trainn_traction_system_4motors_CRH3_ver1/motor module3/Subsystem3/SVPWM1/find section1/not neg1 ==
  In1 : Inport
  Constant2 : Constant  Value=0
  Relational Operator : RelationalOperator  OutDataTypeStr=boolean  RndMeth=Simplest
  Out1 : Outport
  wires:
  Constant2/1 -> Relational Operator/2
  Relational Operator/1 -> Out1/1
  In1/1 -> Relational Operator/1

== system trainn_traction_system_4motors_CRH3_ver1/motor module4/电机控制模块/SVPWM/find section1/>=0? ==
  In1 : Inport
  Constant2 : Constant  Value=0
  Relational Operator : RelationalOperator  OutDataTypeStr=boolean  RndMeth=Simplest
  Out1 : Outport
  wires:
  In1/1 -> Relational Operator/1
  Relational Operator/1 -> Out1/1
  Constant2/1 -> Relational Operator/2

== system trainn_traction_system_4motors_CRH3_ver1/motor module4/电机控制模块/SVPWM/find section1/not neg ==
  In1 : Inport
  Constant2 : Constant  Value=0
  Relational Operator : RelationalOperator  OutDataTypeStr=boolean  RndMeth=Simplest
  Out1 : Outport
  wires:
  Constant2/1 -> Relational Operator/2
  Relational Operator/1 -> Out1/1
  In1/1 -> Relational Operator/1

== system trainn_traction_system_4motors_CRH3_ver1/motor module4/电机控制模块/SVPWM/find section1/not neg1 ==
  In1 : Inport
  Constant2 : Constant  Value=0
  Relational Operator : RelationalOperator  OutDataTypeStr=boolean  RndMeth=Simplest
  Out1 : Outport
  wires:
  In1/1 -> Relational Operator/1
  Relational Operator/1 -> Out1/1
  Constant2/1 -> Relational Operator/2

== system trainn_traction_system_4motors_CRH3_ver1/motor module4/电机控制模块/SVPWM1/find section1/>=0? ==
  In1 : Inport
  Constant2 : Constant  Value=0
  Relational Operator : RelationalOperator  OutDataTypeStr=boolean  RndMeth=Simplest
  Out1 : Outport
  wires:
  Constant2/1 -> Relational Operator/2
  Relational Operator/1 -> Out1/1
  In1/1 -> Relational Operator/1

== system trainn_traction_system_4motors_CRH3_ver1/motor module4/电机控制模块/SVPWM1/find section1/not neg ==
  In1 : Inport
  Constant2 : Constant  Value=0
  Relational Operator : RelationalOperator  OutDataTypeStr=boolean  RndMeth=Simplest
  Out1 : Outport
  wires:
  In1/1 -> Relational Operator/1
  Relational Operator/1 -> Out1/1
  Constant2/1 -> Relational Operator/2

== system trainn_traction_system_4motors_CRH3_ver1/motor module4/电机控制模块/SVPWM1/find section1/not neg1 ==
  In1 : Inport
  Constant2 : Constant  Value=0
  Relational Operator : RelationalOperator  OutDataTypeStr=boolean  RndMeth=Simplest
  Out1 : Outport
  wires:
  Constant2/1 -> Relational Operator/2
  Relational Operator/1 -> Out1/1
  In1/1 -> Relational Operator/1

== matlab function trainn_traction_system_4motors_CRH3_ver1/motor module2/Subsystem2/SVPWM/find section1/get section ==
  data: u input; y output
function y = fcn(u)
switch u
    case 5
        y = 1;
    case 7
        y = 2; 
    case 6
        y = 3;
    case 2
        y = 4;
    case 0
        y = 5;
    case 1
        y = 6;
    otherwise
        y = 0;
end

== matlab function trainn_traction_system_4motors_CRH3_ver1/motor module1/Subsystem1/SVPWM/ Gen Gate ==
  data: t input; t0 input; Ts input; T0 input; T1 input; T2 input; sec input; g output
function g = fcn( t, t0,  Ts, T0, T1, T2, sec)
% T0 = params(1);
% T1 = params(2);
% T2 = params(3);
% sec = params(4);
dt = t - t0;



t_left1 = T0/4;
t_right1 = Ts - T0/4;

t_left2_odd_sec = t_left1 + T1/2;
t_left2_eve_sec = t_left1 + T2/2;
t_left3 = T0/4 + T1/2 + T2/2;
t_right3 = 3*T0/4 + T1/2 + T2/2;
t_right2_odd_sec = Ts - T0/4 - T1/2;
t_right2_eve_sec = Ts - T0/4 - T2/2;


gA = 0;
gB = 0;
gC = 0;

switch sec
    case 1
        if(dt >= t_left1 && dt <= t_right1)
            gA = 1;
        else
            gA = 0;
        end
        if(dt >= t_left2_odd_sec && dt <= t_right2_odd_sec)
            gB = 1;
        else
            gB = 0;
        end
        if(dt >= t_left3 && dt <= t_right3)
            gC = 1;
        else
            gC = 0;
        end
    case 2
        if(dt >= t_left1 && dt <= t_right1)
            gB = 1;
        else
            gB = 0;
        end
        if(dt >= t_left2_eve_sec && dt <= t_right2_eve_sec)
            gA = 1;
        else
            gA = 0;
        end
        if(dt >= t_left3 && dt <= t_right3)
            gC = 1;
        else
            gC = 0;
        end
    case 3
        if(dt >= t_left1 && dt <= t_right1)
            gB = 1;
        else
            gB = 0;
        end
        if(dt >= t_left2_odd_sec && dt <= t_right2_odd_sec)
            gC = 1;
        else
            gC = 0;
        end
        if(dt >= t_left3 && dt <= t_right3)
            gA = 1;
        else
            gA = 0;
        end
    case 4
        if(dt >= t_left1 && dt <= t_right1)
            gC = 1;
        else
            gC = 0;
        end
        if(dt >= t_left2_eve_sec && dt <= t_right2_eve_sec)
            gB = 1;
        else
            gB = 0;
        end
        if(dt >= t_left3 && dt <= t_right3)
            gA = 1;
        else
            gA = 0;
        end
    case 5
        if(dt >= t_left1 && dt <= t_right1)
            gC = 1;
        else
            gC = 0;
        end
        if(dt >= t_left2_odd_sec && dt <= t_right2_odd_sec)
            gA = 1;
        else
            gA = 0;
        end
        if(dt >= t_left3 && dt <= t_right3)
            gB = 1;
        else
            gB = 0;
        end
    case 6
        if(dt > t_left1 && dt < t_right1)
            gA = 1;
        else
            gA = 0;
        end
        if(dt > t_left2_eve_sec && dt < t_right2_eve_sec)
            gC = 1;
        else
            gC = 0;
        end
        if(dt > t_left3 && dt < t_right3)
            gB = 1;
        else
            gB = 0;
        end    
end
g = [gA; 1-gA; gB; 1-gB; gC; 1-gC];

== matlab function trainn_traction_system_4motors_CRH3_ver1/motor module1/Subsystem1/SVPWM/MATLAB Function1 ==
  data: old_t0 input; t input; trigger input; T0 input; new_t0 output; newT0 output; T1 input; T2 input; sec input; oldT0 input; oldT1 input; oldT2 input; oldSec input; newT1 output; newT2 output; newSec output
% function [new_t0, newT] = fcn( old_t0,  t, trigger, T, oldT)
function [new_t0, newT0, newT1, newT2, newSec] = fcn( old_t0,  t, trigger, T0, T1, T2, sec, oldT0, oldT1, oldT2, oldSec)
if(trigger)
    newT0 = T0;
    newT1 = T1;
    newT2 = T2;
    newSec = sec;
    new_t0 = t;
else
    new_t0 = old_t0;
    newT0 = oldT0;
    newT1 = oldT1;
    newT2 = oldT2;
    newSec = oldSec;
end

== matlab function trainn_traction_system_4motors_CRH3_ver1/motor module1/Subsystem1/SVPWM/MATLAB Function3 ==
  data: Udc input; T0 output; Ualpha input; Ubeta input; Ts input; sec input; T1 output; T2 output

function [T0, T1, T2] = fcn( Udc, Ualpha, Ubeta,  Ts, sec)
co = cos((sec-1)*pi/3);
si = sin((sec-1)*pi/3);

Ualpha_ = Ualpha*co + Ubeta*si;
Ubeta_ = -Ualpha*si + Ubeta*co;


T2 = sqrt(3)*Ubeta_/Udc*Ts;
T1 = ( 3*Ualpha_ - sqrt(3)* Ubeta_)/2/Udc*Ts;
T0 = Ts - T1 - T2;

== matlab function trainn_traction_system_4motors_CRH3_ver1/motor module1/Subsystem1/SVPWM/find section1/get section ==
  data: u input; y output
function y = fcn(u)
switch u
    case 5
        y = 1;
    case 7
        y = 2; 
    case 6
        y = 3;
    case 2
        y = 4;
    case 0
        y = 5;
    case 1
        y = 6;
    otherwise
        y = 0;
end

== matlab function trainn_traction_system_4motors_CRH3_ver1/motor module3/Subsystem3/SVPWM/ Gen Gate ==
  data: t input; t0 input; Ts input; T0 input; T1 input; T2 input; sec input; g output
function g = fcn( t, t0,  Ts, T0, T1, T2, sec)
% T0 = params(1);
% T1 = params(2);
% T2 = params(3);
% sec = params(4);
dt = t - t0;



t_left1 = T0/4;
t_right1 = Ts - T0/4;

t_left2_odd_sec = t_left1 + T1/2;
t_left2_eve_sec = t_left1 + T2/2;
t_left3 = T0/4 + T1/2 + T2/2;
t_right3 = 3*T0/4 + T1/2 + T2/2;
t_right2_odd_sec = Ts - T0/4 - T1/2;
t_right2_eve_sec = Ts - T0/4 - T2/2;


gA = 0;
gB = 0;
gC = 0;

switch sec
    case 1
        if(dt >= t_left1 && dt <= t_right1)
            gA = 1;
        else
            gA = 0;
        end
        if(dt >= t_left2_odd_sec && dt <= t_right2_odd_sec)
            gB = 1;
        else
            gB = 0;
        end
        if(dt >= t_left3 && dt <= t_right3)
            gC = 1;
        else
            gC = 0;
        end
    case 2
        if(dt >= t_left1 && dt <= t_right1)
            gB = 1;
        else
            gB = 0;
        end
        if(dt >= t_left2_eve_sec && dt <= t_right2_eve_sec)
            gA = 1;
        else
            gA = 0;
        end
        if(dt >= t_left3 && dt <= t_right3)
            gC = 1;
        else
            gC = 0;
        end
    case 3
        if(dt >= t_left1 && dt <= t_right1)
            gB = 1;
        else
            gB = 0;
        end
        if(dt >= t_left2_odd_sec && dt <= t_right2_odd_sec)
            gC = 1;
        else
            gC = 0;
        end
        if(dt >= t_left3 && dt <= t_right3)
            gA = 1;
        else
            gA = 0;
        end
    case 4
        if(dt >= t_left1 && dt <= t_right1)
            gC = 1;
        else
            gC = 0;
        end
        if(dt >= t_left2_eve_sec && dt <= t_right2_eve_sec)
            gB = 1;
        else
            gB = 0;
        end
        if(dt >= t_left3 && dt <= t_right3)
            gA = 1;
        else
            gA = 0;
        end
    case 5
        if(dt >= t_left1 && dt <= t_right1)
            gC = 1;
        else
            gC = 0;
        end
        if(dt >= t_left2_odd_sec && dt <= t_right2_odd_sec)
            gA = 1;
        else
            gA = 0;
        end
        if(dt >= t_left3 && dt <= t_right3)
            gB = 1;
        else
            gB = 0;
        end
    case 6
        if(dt > t_left1 && dt < t_right1)
            gA = 1;
        else
            gA = 0;
        end
        if(dt > t_left2_eve_sec && dt < t_right2_eve_sec)
            gC = 1;
        else
            gC = 0;
        end
        if(dt > t_left3 && dt < t_right3)
            gB = 1;
        else
            gB = 0;
        end    
end
g = [gA; 1-gA; gB; 1-gB; gC; 1-gC];

== matlab function trainn_traction_system_4motors_CRH3_ver1/motor module3/Subsystem3/SVPWM/MATLAB Function1 ==
  data: old_t0 input; t input; trigger input; T0 input; new_t0 output; newT0 output; T1 input; T2 input; sec input; oldT0 input; oldT1 input; oldT2 input; oldSec input; newT1 output; newT2 output; newSec output
% function [new_t0, newT] = fcn( old_t0,  t, trigger, T, oldT)
function [new_t0, newT0, newT1, newT2, newSec] = fcn( old_t0,  t, trigger, T0, T1, T2, sec, oldT0, oldT1, oldT2, oldSec)
if(trigger)
    newT0 = T0;
    newT1 = T1;
    newT2 = T2;
    newSec = sec;
    new_t0 = t;
else
    new_t0 = old_t0;
    newT0 = oldT0;
    newT1 = oldT1;
    newT2 = oldT2;
    newSec = oldSec;
end

== matlab function trainn_traction_system_4motors_CRH3_ver1/motor module3/Subsystem3/SVPWM/MATLAB Function3 ==
  data: Udc input; T0 output; Ualpha input; Ubeta input; Ts input; sec input; T1 output; T2 output

function [T0, T1, T2] = fcn( Udc, Ualpha, Ubeta,  Ts, sec)
co = cos((sec-1)*pi/3);
si = sin((sec-1)*pi/3);

Ualpha_ = Ualpha*co + Ubeta*si;
Ubeta_ = -Ualpha*si + Ubeta*co;


T2 = sqrt(3)*Ubeta_/Udc*Ts;
T1 = ( 3*Ualpha_ - sqrt(3)* Ubeta_)/2/Udc*Ts;
T0 = Ts - T1 - T2;

== matlab function trainn_traction_system_4motors_CRH3_ver1/motor module3/Subsystem3/SVPWM/find section1/get section ==
  data: u input; y output
function y = fcn(u)
switch u
    case 5
        y = 1;
    case 7
        y = 2; 
    case 6
        y = 3;
    case 2
        y = 4;
    case 0
        y = 5;
    case 1
        y = 6;
    otherwise
        y = 0;
end

== matlab function trainn_traction_system_4motors_CRH3_ver1/MATLAB Function ==
  data: nr1 input; nr1_ output; nr2_ output; nr3_ output; nr2 input; nr3 input; nr4 input; nr4_ output
function [nr1_, nr2_, nr3_, nr4_] = fcn(nr1, nr2, nr3, nr4)

nr1_  = nr1 + 0.3*(nr1 - nr2) + 0.11*(nr1 - nr3) + 0.07*(nr1 - nr4);
nr2_  = nr2 + 0.3*(nr2 - nr1) + 0.09*(nr2 - nr3) + 0.11*(nr2 - nr4);
nr3_  = nr3 + 0.11*(nr3 - nr1) + 0.09*(nr3 - nr2) + 0.3*(nr3 - nr4);
nr4_  = nr4 + 0.07*(nr4 - nr1) + 0.11*(nr4 - nr2) + 0.3*(nr4 - nr3);

% nr1_  = nr1 + 0.3*(nr1 - nr2) + 0.3*(nr1 - nr3) + 0.3*(nr1 - nr4);
% nr2_  = nr2 + 0.3*(nr2 - nr1) + 0.3*(nr2 - nr3) + 0.3*(nr2 - nr4);
% nr3_  = nr3 + 0.3*(nr3 - nr1) + 0.3*(nr3 - nr2) + 0.3*(nr3 - nr4);
% nr4_  = nr4 + 0.3*(nr4 - nr1) + 0.3*(nr4 - nr2) + 0.3*(nr4 - nr3);
